simulink model "pr513_am_ssb"  (R2018b)
settings: Solver=VariableStepAuto  StartTime=0.0  StopTime=100*time_span  RelTol=1e-3  EnableMultiTasking=on
PreLoadFcn:
  | pr51setup;
values from neighbouring files (symbols this model uses):
  filter_order = 1000    [pr51setup.m]
  fs = 500e3    (= 500000)    [pr51setup.m]
undefined symbols (not defined in the file or in its folder): bband1, bband2, bband3, bband4, carrier, fdesignblkfcn, gcbh, single
libraries: dspsrcs4 x7
CloseFcn:
  | clear all;
settings Model: Creator=GRIHA  LastModifiedBy=Григорий Фокин
settings DataIOCC: LimitDataPoints=on
settings OptimizationCC: LifeSpan=inf
settings DebuggingCC: AllowSymbolicDim=off  SFUnexpectedBacktrackingDiag=warning  SFNoUnconditionalDefaultTransitionDiag=warning  SFExecutionAtInitializationDiag=none
settings ModelReferenceCC: PropagateSignalLabelsOutOfModel=off
settings SFSimCC: SimUseLocalCustomCode=off
settings RTWCC: RTWUseLocalCustomCode=off
settings CodeAppCC: StateflowObjectComments=on
settings GRTTargetCC: TargetLangStandard=C89/C90 (ANSI)
settings ConfigComp: CovMetricSettings=dw  CovHtmlReporting=on  CovSaveCumulativeToWorkspaceVar=on  CovSaveSingleToWorkspaceVar=on  CovExternalEMLEnable=off

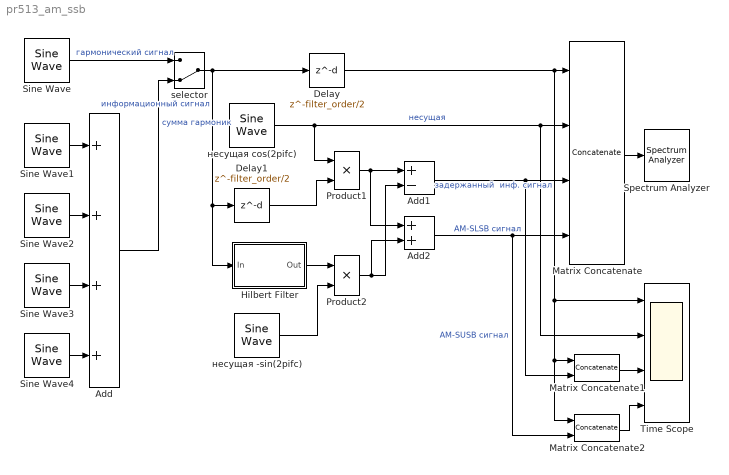
== system pr513_am_ssb ==
  Add : Sum  Inputs=++++
  Add1 : Sum  Inputs=+-
  Add2 : Sum
  Delay : Delay  DelayLength=filter_order/2  InitialCondition=0
  Delay1 : Delay  DelayLength=filter_order/2  InitialCondition=0
  Hilbert Filter : Subsystem  DialogController=fdesignblkfcn  InitFcn=fdesignblkfcn(gcbh, {'InitFcn'});  mask(Hilbert Filter){}
      mask help: Design a Hilbert filter
      settings: CopyFcn=fdesignblkfcn(gcbh, {'CopyFcn'});
      mask Help: helpview(mapfilelocation('dsp'), 'dsphilbertfilter');
      mask Display: disp('Hilbert')
  Matrix Concatenate : Concatenate  NumInputs=4  Mode=Multidimensional array  ConcatenateDimension=2
  Matrix Concatenate1 : Concatenate  Mode=Multidimensional array  ConcatenateDimension=2
  Matrix Concatenate2 : Concatenate  Mode=Multidimensional array  ConcatenateDimension=2
  Product1 : Product
  Product2 : Product
  Sine Wave : dspsrcs4/Sine Wave  Amplitude=single.Ai  Frequency=single.fi  Phase=single.ph  SampleMode=Discrete  OutComplex=Real  CompMethod=Trigonometric fcn  TableSize=Speed  SampleTime=1/fs  SamplesPerFrame=1  ResetState=Restart at time zero  OutputFrames=off  dataType=double  wordLen=16  udDataType=sfix(16)  fracBitsMode=Best precision  numFracBits=15  OutDataTypeStr=double  LastOutDataTypeStr=double
  Sine Wave1 : dspsrcs4/Sine Wave  Amplitude=bband1.Ai  Frequency=bband1.fi  Phase=bband1.ph  SampleMode=Discrete  OutComplex=Real  CompMethod=Trigonometric fcn  TableSize=Speed  SampleTime=1/fs  SamplesPerFrame=1  ResetState=Restart at time zero  OutputFrames=off  dataType=double  wordLen=16  udDataType=sfix(16)  fracBitsMode=Best precision  numFracBits=15  OutDataTypeStr=double  LastOutDataTypeStr=double
  Sine Wave2 : dspsrcs4/Sine Wave  Amplitude=bband2.Ai  Frequency=bband2.fi  Phase=bband2.ph  SampleMode=Discrete  OutComplex=Real  CompMethod=Trigonometric fcn  TableSize=Speed  SampleTime=1/fs  SamplesPerFrame=1  ResetState=Restart at time zero  OutputFrames=off  dataType=double  wordLen=16  udDataType=sfix(16)  fracBitsMode=Best precision  numFracBits=15  OutDataTypeStr=double  LastOutDataTypeStr=double
  Sine Wave3 : dspsrcs4/Sine Wave  Amplitude=bband3.Ai  Frequency=bband3.fi  Phase=bband3.ph  SampleMode=Discrete  OutComplex=Real  CompMethod=Trigonometric fcn  TableSize=Speed  SampleTime=1/fs  SamplesPerFrame=1  ResetState=Restart at time zero  OutputFrames=off  dataType=double  wordLen=16  udDataType=sfix(16)  fracBitsMode=Best precision  numFracBits=15  OutDataTypeStr=double  LastOutDataTypeStr=double
  Sine Wave4 : dspsrcs4/Sine Wave  Amplitude=bband4.Ai  Frequency=bband4.fi  Phase=bband4.ph  SampleMode=Discrete  OutComplex=Real  CompMethod=Trigonometric fcn  TableSize=Speed  SampleTime=1/fs  SamplesPerFrame=1  ResetState=Restart at time zero  OutputFrames=off  dataType=double  wordLen=16  udDataType=sfix(16)  fracBitsMode=Best precision  numFracBits=15  OutDataTypeStr=double  LastOutDataTypeStr=double
  Spectrum Analyzer : SpectrumAnalyzer
  Time Scope : Scope  NumInputPorts=4
  selector : ManualSwitch  CurrentSetting=0
  несущая cos(2pifc) : dspsrcs4/Sine Wave  Amplitude=carrier.Ac  Frequency=carrier.fc  Phase=carrier.ph  SampleMode=Discrete  OutComplex=Real  CompMethod=Trigonometric fcn  TableSize=Speed  SampleTime=1/fs  SamplesPerFrame=1  ResetState=Restart at time zero  OutputFrames=off  dataType=double  wordLen=16  udDataType=sfix(16)  fracBitsMode=Best precision  numFracBits=15  OutDataTypeStr=double  LastOutDataTypeStr=double
  несущая -sin(2pifc) : dspsrcs4/Sine Wave  Amplitude=carrier.Ac  Frequency=carrier.fc  Phase=carrier.ph+(pi/2)  SampleMode=Discrete  OutComplex=Real  CompMethod=Trigonometric fcn  TableSize=Speed  SampleTime=1/fs  SamplesPerFrame=1  ResetState=Restart at time zero  OutputFrames=off  dataType=double  wordLen=16  udDataType=sfix(16)  fracBitsMode=Best precision  numFracBits=15  OutDataTypeStr=double  LastOutDataTypeStr=double
  wires:
  Sine Wave1/1 -> Add/1
  Sine Wave2/1 -> Add/2
  Sine Wave3/1 -> Add/3
  Sine Wave4/1 -> Add/4
  Sine Wave/1 -> selector/1  "гармонический сигнал"
  Add/1 -> selector/2  "сумма гармоник"
  selector/1 -> Hilbert Filter/1(In), Delay1/1, Delay/1  "информационный сигнал"
  несущая cos(2pifc)/1 -> Product1/1, Time Scope/2, Matrix Concatenate/2  "несущая"
  Matrix Concatenate/1 -> Spectrum Analyzer/1
  Delay/1 -> Matrix Concatenate2/1, Matrix Concatenate1/1, Time Scope/1, Matrix Concatenate/1  "задержанный  инф. сигнал"
  Delay1/1 -> Product1/2
  Hilbert Filter/1(Out) -> Product2/1
  несущая -sin(2pifc)/1 -> Product2/2
  Product1/1 -> Add2/1, Add1/1
  Product2/1 -> Add1/2, Add2/2
  Add1/1 -> Matrix Concatenate1/2, Matrix Concatenate/3  "AM-SLSB сигнал"
  Add2/1 -> Matrix Concatenate2/2, Matrix Concatenate/4  "AM-SUSB сигнал"
  Matrix Concatenate1/1 -> Time Scope/3
  Matrix Concatenate2/1 -> Time Scope/4

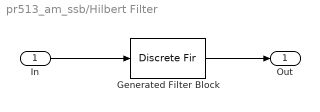
== system pr513_am_ssb/Hilbert Filter ==
  In : Inport
  Generated Filter Block : DiscreteFir  Tag=BlockMethodSubSystem  Coefficients=[-1.340315280530221e-12 -0.15532194863759521 9.985909825208318e-13 -0.0012125629072069488 5.580618670101296e-14 -0.0012182496068171844 -1.7598529487556406e-14 -0.0012245344503327704 -4.5516283990885644e-14 -0.0012314293369682372 -3.0538739237332598e-14 -0.0012393260537777451 5.9098395590415978e-14 -0.0012472558880338713 -3.5026668228246942e-14 -0.0012564291405026129 5.340919020909386e-14 -0.0012661979243051569 -3.4744806766751259e-14 -0.0012766892969970911 -3.6520665714358337e-14 -0.0012880682500244767 5.5870281420838448e-14 -0.0012996718338555979 -2.7526916028471199e-14 -0.0013126692223279779 5.2576673923384309e-14 -0.0013261803834903052 -3.6574928915612234e-14 -0.0013405459376820694 5.1545509080176805e-14 -0.0013558098056489776 -3.3878337403234108e-14 -0.001038627041047846 -1.2537343135498253e-14 -0.0013030805852580762 -1.5481985806218638e-14 -0.0013098661552599644 4.9376991894322905e-14 -0.001316629853382878 -4.7464413830976019e-14 -0.001323336672594877 5.5702115782242435e-14 -0.0013294519213009615 3.9939335551084879e-14 -0.0013360348384328091 -9.255247373655175e-14 -0.0013416852810341773 4.2957846145765286e-14 -0.0013469961212466686 -2.2293560596590299e-14 -0.0013517897437340665 5.2747895103173726e-14 -0.0013557657170180093 -2.9458590568533263e-14 -0.0013595423457086753 5.0413880592718169e-14 -0.0013618093600573644 -1.0247558346820826e-13 -0.0013633025167925084 6.1234079738680301e-14 -0.0013635785431320713 -2.4976971780873197e-14 -0.0013624223367134647 6.5374370154517188e-15 -0.0014615636337156346 7.7994132914318003e-14 -0.0014068877996473717 -2.2147599328559654e-14 -0.0014135446008163299 4.3357080249492394e-14 -0.001420147353961454 -8.7450233682022e-14 -0.0014266760065151374 4.9888535427040014e-14 -0.0014337355970166499 -2.8962861805665024e-14 -0.0014401206768379637 4.80629118798732e-14 -0.0014473236801961775 -2.3304333860145389e-14 -0.0014547690940238667 3.8555321114775796e-14 -0.0014626205928935931 -3.3609263515055093e-15 -0.0014712594853731886 -3.9086426630927885e-14 -0.0014800943825541424 5.2815646705616778e-14 -0.0014905159071512131 -3.7589993915742923e-14 -0.0015019474074122741 6.6667006943053202e-14 -0.0015149339027082931 -4.4731664404696151e-14 -0.0015298890464983117 7.7128898836568718e-15 -0.0014939998792549147 -3.9358236647686242e-14 -0.0015270246531944309 4.5256497761291561e-14 -0.0015352437426034982 -2.2840960019125482e-14 -0.0015436878006642729 4.3942863284614687e-14 -0.001552448101765691 4.0172439146170615e-14 -0.0015608607198753788 -1.1392934590613626e-14 -0.0015703050025894782 -3.2864909209181014e-14 -0.0015792358518389449 -2.1054634375052654e-14 -0.0015882336228809635 3.76183792437466e-14 -0.0015971909643308635 -1.2526380838415727e-14 -0.0016056899964933535 4.535749754161709e-14 -0.0016143261307561829 -2.9657355146762787e-14 -0.0016216744153361162 -1.5452600717768797e-14 -0.0016281714151666904 -1.84262816213811e-14 -0.0016331837656622383 5.0951059027823861e-14 -0.0016360942438922166 2.4784089244160161e-14 -0.0016709620533106317 -1.2621632494898273e-14 -0.0016677918798535529 4.2813522163967964e-14 -0.0016773823675499955 -2.7137730759384079e-14 -0.0016869558504577498 -1.3470968713262251e-14 -0.001696358908709783 -1.90611269292699e-14 -0.001706333573487484 4.2629885977692552e-14 -0.0017153215891418938 -2.0319774036487996e-14 -0.0017249144861857246 4.8940950493562005e-14 -0.001734529172283672 -3.5834220493160429e-14 -0.0017442008747821092 2.8440672505143517e-15 -0.0017543615755926112 3.5948837720781492e-14 -0.0017643946544740885 -2.1826878296552972e-14 -0.0017757329954317669 4.1198802014925922e-14 -0.0017880661760862893 -2.1354266199723356e-14 -0.0018021115484145867 3.3218359806976189e-14 -0.0018187012853339013 -4.9407340091085074e-14 -0.0018131900421778369 2.2873657484191211e-14 -0.0018315054300579447 -1.743755309112808e-14 -0.0018426232130543951 5.1454560449676096e-14 -0.0018539338346847956 -2.0482863275773403e-14 -0.0018656535963899046 5.8567260554174594e-14 -0.0018769474551341148 3.6926975744851702e-14 ...(+18817 chars)]  InputProcessing=Columns as channels (frame based)
  Out : Outport
  wires:
  Generated Filter Block/1 -> Out/1
  In/1 -> Generated Filter Block/1
